simulink model "modelo_pendulo"  (R2018a)
settings: Solver=ode45  StartTime=0.0  StopTime=10.0  RelTol=1e-3  EnableMultiTasking=on
values from neighbouring files (symbols this model uses):
  A = [0 1 0 0; 20.601 0 0 0; 0 0 0 1; -0.4905 0 0 0]    [pendulo.m]
  B = [0; -1; 0; 0.5]    [pendulo.m]
  C = [0 0 1 0]    [pendulo.m]
  D = zeros(size(C*B))    [pendulo.m]
  K = [157.6336 35.3733 56.0652 36.7466]    [pendulo.m]
  kI = 50.9684    [pendulo.m]
libraries: simulink x1
settings Model: Creator=Prof.DanielFernandes  LastModifiedBy=wesle
settings DataIOCC: LimitDataPoints=on  SaveFormat=Array
settings OptimizationCC: LifeSpan=inf
settings DebuggingCC: UnderspecifiedInitializationDetection=Classic  MergeDetectMultiDrivingBlocksExec=none  SolverPrmCheckMsg=warning  SFUnexpectedBacktrackingDiag=warning  SFNoUnconditionalDefaultTransitionDiag=warning  SFExecutionAtInitializationDiag=none
settings HardwareCC: ProdBitPerPointer=32  ProdBitPerSizeT=32  ProdBitPerPtrDiffT=32  ProdLargestAtomicFloat=None  ProdIntDivRoundTo=Undefined  ProdEndianess=Unspecified  ProdWordSize=32  ProdHWDeviceType=32-bit Generic
settings ModelReferenceCC: PropagateSignalLabelsOutOfModel=off
settings CodeAppCC: StateflowObjectComments=on
settings GRTTargetCC: TargetLangStandard=C89/C90 (ANSI)  GeneratePreprocessorConditionals=Disable all
settings ConfigComp: CovMetricSettings=dw  CovHtmlReporting=on  CovSaveCumulativeToWorkspaceVar=on  CovSaveSingleToWorkspaceVar=on  CovExternalEMLEnable=off

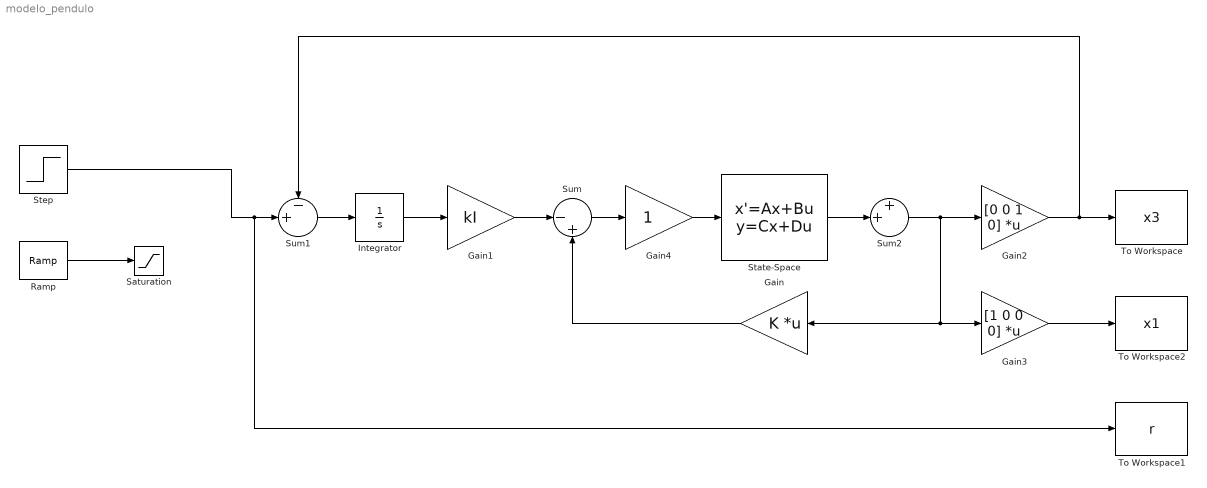
== system modelo_pendulo ==
  Gain : Gain  Gain=K  Multiplication=Matrix(K*u) (u vector)
  Gain1 : Gain  Gain=kI
  Gain2 : Gain  Gain=[0 0 1 0]  Multiplication=Matrix(K*u) (u vector)
  Gain3 : Gain  Gain=[1 0 0 0]  Multiplication=Matrix(K*u) (u vector)
  Gain4 : Gain
  Integrator : Integrator
  Ramp : simulink/Sources/Ramp  slope=1  start=0  InitialOutput=0
  Saturation : Saturate  UpperLimit=2  LowerLimit=0
  State-Space : StateSpace  A=A  B=B  C=C  D=D  InitialCondition=0
  Step : Step  Time=0  After=1.7  SampleTime=0
  Sum : Sum  Inputs=|-+
  Sum1 : Sum  Inputs=-+|
  Sum2 : Sum  Inputs=++|
  To Workspace : ToWorkspace  VariableName=x3  SampleTime=-1
  To Workspace1 : ToWorkspace  VariableName=r  SampleTime=-1
  To Workspace2 : ToWorkspace  VariableName=x1  SampleTime=-1
  wires:
  Gain/1 -> Sum/2
  Gain1/1 -> Sum/1
  Integrator/1 -> Gain1/1
  Sum1/1 -> Integrator/1
  Gain3/1 -> To Workspace2/1
  Gain4/1 -> State-Space/1
  Sum/1 -> Gain4/1
  Gain2/1 -> Sum1/1, To Workspace/1
  State-Space/1 -> Sum2/2
  Sum2/1 -> Gain3/1, Gain/1, Gain2/1
  Ramp/1 -> Saturation/1
  Step/1 -> To Workspace1/1, Sum1/2
